simulink model "ADCS_Model"  (R2017b)
settings: Solver=FixedStepAuto  StartTime=0.0  StopTime=10000  FixedStep=1  RelTol=1e-3
libraries: sharedTrackingLibrary x3, simulink x1
settings Model: Creator=caspe  LastModifiedBy=caspe

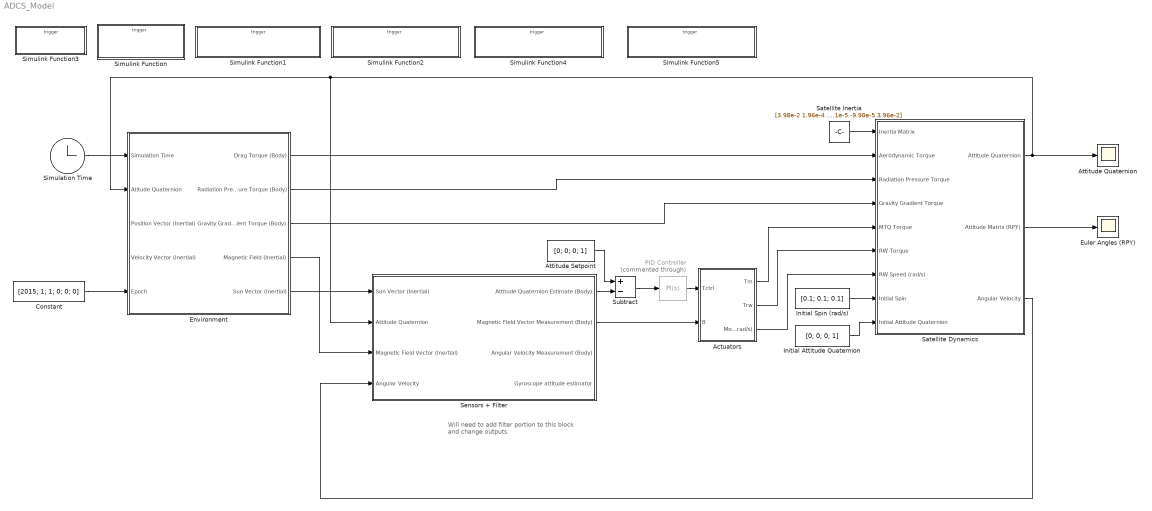
== system ADCS_Model ==
  note: Will need to add filter portion to this block
      | and change outputs.
  Actuators : Subsystem
  Attitude Quaternion : Scope
  Attitude Setpoint : Constant  Value=[0; 0; 0; 1]
  Constant : Constant  Value=[2015; 1; 1; 0; 0; 0]
  Environment : Subsystem
  Euler Angles (RPY) : Scope
  Initial Attitude Quaternion : Constant  Value=[0; 0; 0; 1]
  Initial Spin (rad/s) : Constant  Value=[0.1; 0.1; 0.1]
  PID Controller : simulink/Continuous/PID Controller  Commented=through  Controller=PI  TimeDomain=Continuous-time  SampleTime=-1  IntegratorMethod=Forward Euler  FilterMethod=Forward Euler  Form=Parallel  UseFilter=on  ControllerParametersSource=internal  P=eye(4)  I=eye(4)  D=1.1*eye(4)  N=100  InitialConditionSource=internal  InitialConditionForIntegrator=0  InitialConditionForFilter=0  ExternalReset=none  LimitOutput=off  UpperSaturationLimit=inf  LowerSaturationLimit=-inf  LinearizeAsGain=on  AntiWindupMode=none  Kb=1  TrackingMode=off  Kt=1  PParamMin=[]  PParamMax=[]  IParamMin=[]  IParamMax=[]  DParamMin=[]  DParamMax=[]  NParamMin=[]  NParamMax=[]  KbParamMin=[]  KbParamMax=[]  KtParamMin=[]  KtParamMax=[]  POutMin=[]  POutMax=[]  IOutMin=[]  IOutMax=[]  DOutMin=[]  DOutMax=[]  NOutMin=[]  NOutMax=[]  KbOutMin=[]  KbOutMax=[]  KtOutMin=[]  KtOutMax=[]  IntegratorOutMin=[]  IntegratorOutMax=[]  FilterOutMin=[]  FilterOutMax=[]  SumOutMin=[]  SumOutMax=[]  SumI1OutMin=[]  SumI1OutMax=[]  SumI2OutMin=[]  SumI2OutMax=[]  SumI3OutMin=[]  SumI3OutMax=[]  SumDOutMin=[]  SumDOutMax=[]  SaturationOutMin=[]  SaturationOutMax=[]  IntegratorContinuousStateAttributes=''  IntegratorStateMustResolveToSignalObject=off  IntegratorRTWStateStorageClass=Auto  FilterContinuousStateAttributes=''  FilterStateMustResolveToSignalObject=off  FilterRTWStateStorageClass=Auto  DifferentiatorICPrevScaledInput=0  DifferentiatorOutMin=[]  DifferentiatorOutMax=[]  InitialConditionSetting=State (most efficient)  FilterDiffOutCoefMin=[]  FilterDiffOutCoefMax=[]  SumDenOutMin=[]  SumDenOutMax=[]  SumNumOutMin=[]  SumNumOutMax=[]  ReciprocalOutMin=[]  ReciprocalOutMax=[]  DivideOutMin=[]  DivideOutMax=[]  TunerSelectOption=Transfer Function Based (PID Tuner App)
  Satellite Dynamics : Subsystem
  Satellite Inertia : Constant  Value=[3.98e-2 1.96e-4 2.1e-5; 1.96e-4 7.54e-3 -9.98e-5; 2.1e-5 -9.98e-5 3.96e-2]  VectorParams1D=off
  Sensors + Filter : Subsystem
  Simulation Time : Clock
  Simulink Function : Subsystem  TreatAsAtomicUnit=on
  Simulink Function1 : Subsystem  TreatAsAtomicUnit=on
  Simulink Function2 : Subsystem  TreatAsAtomicUnit=on
  Simulink Function3 : Subsystem  TreatAsAtomicUnit=on
  Simulink Function4 : Subsystem  TreatAsAtomicUnit=on
  Simulink Function5 : Subsystem  TreatAsAtomicUnit=on
  Subtract : Sum  Inputs=+-
  wires:
  Simulation Time/1 -> Environment/1(Simulation Time)
  Environment/4(Magnetic Field (Inertial)) -> Sensors + Filter/3(Magnetic Field Vector (Inertial))
  Environment/5(Sun Vector (Inertial)) -> Sensors + Filter/1(Sun Vector (Inertial))
  Satellite Inertia/1 -> Satellite Dynamics/1(Inertia Matrix)
  Environment/1(Drag Torque (Body)) -> Satellite Dynamics/2(Aerodynamic Torque)
  Environment/2(Radiation Pressure Torque (Body)) -> Satellite Dynamics/3(Radiation Pressure Torque)
  Environment/3(Gravity Gradient Torque (Body)) -> Satellite Dynamics/4(Gravity Gradient Torque)
  Satellite Dynamics/3(Angular Velocity) -> Sensors + Filter/4(Angular Velocity)
  Satellite Dynamics/1(Attitude Quaternion) -> Attitude Quaternion/1, Sensors + Filter/2(Attitude Quaternion), Environment/2(Atitude Quaternion)
  Initial Spin (rad/s)/1 -> Satellite Dynamics/8(Initial Spin)
  Initial Attitude Quaternion/1 -> Satellite Dynamics/9(Initial Attitude Quaternion)
  Constant/1 -> Environment/5(Epoch)
  Satellite Dynamics/2(Attitude Matrix (RPY)) -> Euler Angles (RPY)/1
  Subtract/1 -> PID Controller/1
  Attitude Setpoint/1 -> Subtract/1
  Sensors + Filter/1(Attitude Quaternion Estimate (Body)) -> Subtract/2
  PID Controller/1 -> Actuators/1(Tctrl)
  Sensors + Filter/2(Magnetic Field Vector Measurement (Body)) -> Actuators/2(B)
  Actuators/2(Trw) -> Satellite Dynamics/6(RW Torque)
  Actuators/1(Tm) -> Satellite Dynamics/5(MTQ Torque)
  Actuators/3(Momentum wheel speed (rad/s)) -> Satellite Dynamics/7(RW Speed (rad/s))

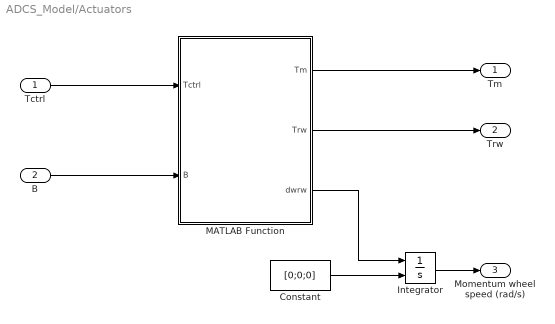
== system ADCS_Model/Actuators ==
  Tctrl : Inport
  B : Inport  Port=2
  Constant : Constant  Value=[0;0;0]
  Integrator : Integrator  InitialConditionSource=external
  MATLAB Function : MATLAB Function  TreatAsAtomicUnit=on
  Tm : Outport
  Trw : Outport  Port=2
  Momentum wheel speed (rad/s) : Outport  Port=3
  wires:
  Tctrl/1 -> MATLAB Function/1(Tctrl)
  B/1 -> MATLAB Function/2(B)
  MATLAB Function/1(Tm) -> Tm/1
  MATLAB Function/2(Trw) -> Trw/1
  MATLAB Function/3(dwrw) -> Integrator/1
  Integrator/1 -> Momentum wheel speed (rad/s)/1
  Constant/1 -> Integrator/2

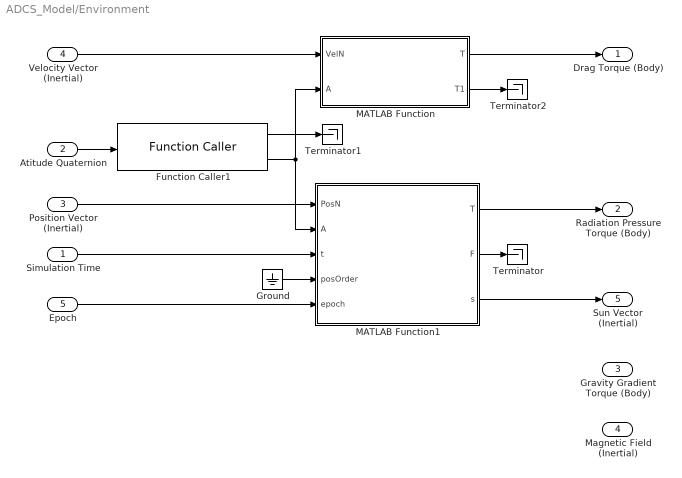
== system ADCS_Model/Environment ==
  Simulation Time : Inport
  Atitude Quaternion : Inport  Port=2
  Position Vector (Inertial) : Inport  Port=3
  Velocity Vector (Inertial) : Inport  Port=4
  Epoch : Inport  Port=5
  Function Caller1 : FunctionCaller  FunctionPrototype=[q,A] = quaternionAttitudeMatrix(x)
  Ground : Ground
  MATLAB Function : MATLAB Function  TreatAsAtomicUnit=on
  MATLAB Function1 : MATLAB Function  TreatAsAtomicUnit=on
  Terminator : Terminator
  Terminator1 : Terminator
  Terminator2 : Terminator
  Drag Torque (Body) : Outport
  Radiation Pressure Torque (Body) : Outport  Port=2
  Gravity Gradient Torque (Body) : Outport  Port=3
  Magnetic Field (Inertial) : Outport  Port=4
  Sun Vector (Inertial) : Outport  Port=5
  wires:
  Velocity Vector (Inertial)/1 -> MATLAB Function/1(VelN)
  Atitude Quaternion/1 -> Function Caller1/1
  Simulation Time/1 -> MATLAB Function1/3(t)
  Position Vector (Inertial)/1 -> MATLAB Function1/1(PosN)
  Function Caller1/1 -> Terminator1/1
  Function Caller1/2 -> MATLAB Function1/2(A), MATLAB Function/2(A)
  MATLAB Function/2(T1) -> Terminator2/1
  MATLAB Function/1(T) -> Drag Torque (Body)/1
  Ground/1 -> MATLAB Function1/4(posOrder)
  Epoch/1 -> MATLAB Function1/5(epoch)
  MATLAB Function1/2(F) -> Terminator/1
  MATLAB Function1/3(s) -> Sun Vector (Inertial)/1
  MATLAB Function1/1(T) -> Radiation Pressure Torque (Body)/1

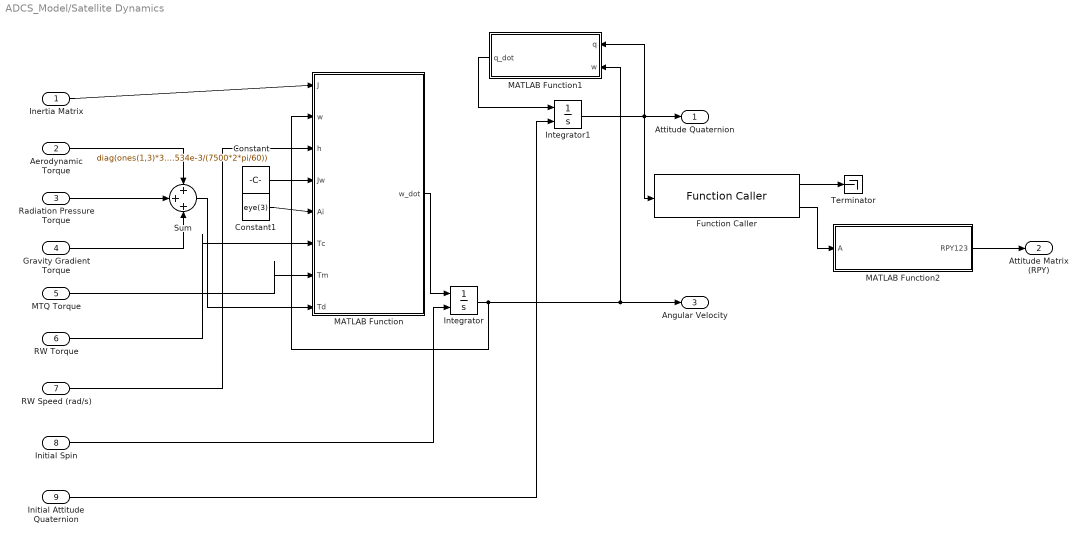
== system ADCS_Model/Satellite Dynamics ==
  Inertia Matrix : Inport
  Aerodynamic Torque : Inport  Port=2
  Radiation Pressure Torque : Inport  Port=3
  Gravity Gradient Torque : Inport  Port=4
  MTQ Torque : Inport  Port=5
  RW Torque : Inport  Port=6
  RW Speed (rad/s) : Inport  Port=7
  Initial Spin : Inport  Port=8
  Initial Attitude Quaternion : Inport  Port=9
  Constant : Constant  Value=diag(ones(1,3)*3.534e-3/(7500*2*pi/60))
  Constant1 : Constant  Value=eye(3)
  Function Caller : FunctionCaller  FunctionPrototype=[q,A] = quaternionAttitudeMatrix(x)
  Integrator : Integrator  InitialConditionSource=external
  Integrator1 : Integrator  InitialConditionSource=external
  MATLAB Function : MATLAB Function  TreatAsAtomicUnit=on
  MATLAB Function1 : MATLAB Function  TreatAsAtomicUnit=on
  MATLAB Function2 : MATLAB Function  TreatAsAtomicUnit=on
  Sum : Sum  Inputs=+++
  Terminator : Terminator
  Attitude Quaternion : Outport
  Attitude Matrix (RPY) : Outport  Port=2
  Angular Velocity : Outport  Port=3
  wires:
  Aerodynamic Torque/1 -> Sum/1
  Radiation Pressure Torque/1 -> Sum/2
  Gravity Gradient Torque/1 -> Sum/3
  RW Torque/1 -> MATLAB Function/6(Tc)
  Integrator/1 -> MATLAB Function/2(w), MATLAB Function1/2(w), Angular Velocity/1
  Initial Spin/1 -> Integrator/2
  MTQ Torque/1 -> MATLAB Function/7(Tm)
  MATLAB Function/1(w_dot) -> Integrator/1
  RW Speed (rad/s)/1 -> MATLAB Function/3(h)
  Inertia Matrix/1 -> MATLAB Function/1(J)
  Sum/1 -> MATLAB Function/8(Td)
  Constant/1 -> MATLAB Function/4(Jw)
  Constant1/1 -> MATLAB Function/5(Ai)
  Initial Attitude Quaternion/1 -> Integrator1/2
  Integrator1/1 -> Function Caller/1, MATLAB Function1/1(q), Attitude Quaternion/1
  MATLAB Function1/1(q_dot) -> Integrator1/1
  Function Caller/1 -> Terminator/1
  Function Caller/2 -> MATLAB Function2/1(A)
  MATLAB Function2/1(RPY123) -> Attitude Matrix (RPY)/1

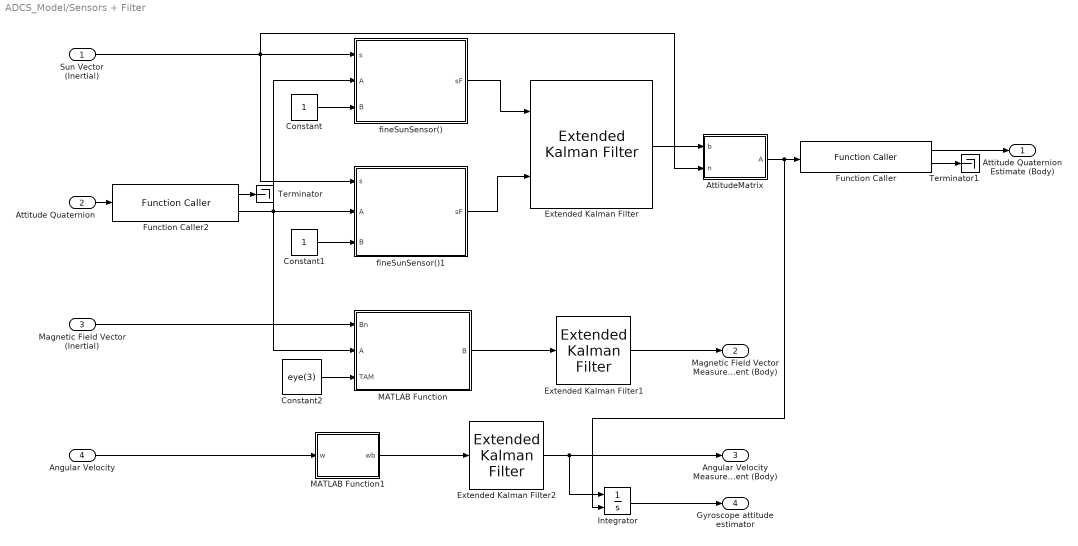
== system ADCS_Model/Sensors + Filter ==
  Sun Vector (Inertial) : Inport
  Attitude Quaternion : Inport  Port=2
  Magnetic Field Vector (Inertial) : Inport  Port=3
  Angular Velocity : Inport  Port=4
  AttitudeMatrix : MATLAB Function  TreatAsAtomicUnit=on
  Constant : Constant
  Constant1 : Constant
  Constant2 : Constant  Value=eye(3)
  Extended Kalman Filter : sharedTrackingLibrary/Extended Kalman Filter  StateTransitionFcn=stateTrans  HasStateTransitionJacobianFcn=off  HasAdditiveProcessNoise=Additive  ProcessNoise=1  HasTimeVaryingProcessNoise=off  HasStateTransitionFcnExtraArgument=0  InitialState=0  InitialStateCovariance=1  MeasurementFcn1=addSunSensorNoise  HasMeasurementJacobianFcn1=off  HasMeasurementEnablePort1=off  HasAdditiveMeasurementNoise1=Additive  MeasurementNoise1=1  HasTimeVaryingMeasurementNoise1=off  HasMeasurementFcnExtraArgument1=0  MeasurementFcn2=addSunSensorNoise  HasMeasurementJacobianFcn2=off  HasMeasurementEnablePort2=off  HasAdditiveMeasurementNoise2=Additive  MeasurementNoise2=1  HasTimeVaryingMeasurementNoise2=off  HasMeasurementFcnExtraArgument2=0  MeasurementFcn3=myMeasurementFcn  HasMeasurementJacobianFcn3=off  HasMeasurementEnablePort3=off  HasAdditiveMeasurementNoise3=Additive  MeasurementNoise3=1  HasTimeVaryingMeasurementNoise3=off  HasMeasurementFcnExtraArgument3=0  MeasurementFcn4=myMeasurementFcn  HasMeasurementJacobianFcn4=off  HasMeasurementEnablePort4=off  HasAdditiveMeasurementNoise4=Additive  MeasurementNoise4=1  HasTimeVaryingMeasurementNoise4=off  HasMeasurementFcnExtraArgument4=0  MeasurementFcn5=myMeasurementFcn  HasMeasurementJacobianFcn5=off  HasMeasurementEnablePort5=off  HasAdditiveMeasurementNoise5=Additive  MeasurementNoise5=1  HasTimeVaryingMeasurementNoise5=off  HasMeasurementFcnExtraArgument5=0  EnableMultirate=off  StateTransitionFcnSampleTime=1  MeasurementFcn1SampleTime=1  MeasurementFcn2SampleTime=1  MeasurementFcn3SampleTime=1  MeasurementFcn4SampleTime=1  MeasurementFcn5SampleTime=1  UseCurrentEstimator=on  OutputStateCovariance=off  DataType=double  SampleTime=1  NumberOfMeasurements=2
      settings: SourceProductName=Control System Toolbox  SourceProductBaseCode=CT
  Extended Kalman Filter1 : sharedTrackingLibrary/Extended Kalman Filter  StateTransitionFcn=stateTrans  HasStateTransitionJacobianFcn=off  HasAdditiveProcessNoise=Additive  ProcessNoise=1  HasTimeVaryingProcessNoise=off  HasStateTransitionFcnExtraArgument=0  InitialState=0  InitialStateCovariance=1  MeasurementFcn1=addTAMNoise  HasMeasurementJacobianFcn1=off  HasMeasurementEnablePort1=off  HasAdditiveMeasurementNoise1=Additive  MeasurementNoise1=1  HasTimeVaryingMeasurementNoise1=off  HasMeasurementFcnExtraArgument1=0  MeasurementFcn2=myMeasurementFcn  HasMeasurementJacobianFcn2=off  HasMeasurementEnablePort2=off  HasAdditiveMeasurementNoise2=Additive  MeasurementNoise2=1  HasTimeVaryingMeasurementNoise2=off  HasMeasurementFcnExtraArgument2=0  MeasurementFcn3=myMeasurementFcn  HasMeasurementJacobianFcn3=off  HasMeasurementEnablePort3=off  HasAdditiveMeasurementNoise3=Additive  MeasurementNoise3=1  HasTimeVaryingMeasurementNoise3=off  HasMeasurementFcnExtraArgument3=0  MeasurementFcn4=myMeasurementFcn  HasMeasurementJacobianFcn4=off  HasMeasurementEnablePort4=off  HasAdditiveMeasurementNoise4=Additive  MeasurementNoise4=1  HasTimeVaryingMeasurementNoise4=off  HasMeasurementFcnExtraArgument4=0  MeasurementFcn5=myMeasurementFcn  HasMeasurementJacobianFcn5=off  HasMeasurementEnablePort5=off  HasAdditiveMeasurementNoise5=Additive  MeasurementNoise5=1  HasTimeVaryingMeasurementNoise5=off  HasMeasurementFcnExtraArgument5=0  EnableMultirate=off  StateTransitionFcnSampleTime=1  MeasurementFcn1SampleTime=1  MeasurementFcn2SampleTime=1  MeasurementFcn3SampleTime=1  MeasurementFcn4SampleTime=1  MeasurementFcn5SampleTime=1  UseCurrentEstimator=on  OutputStateCovariance=off  DataType=double  SampleTime=1  NumberOfMeasurements=1
      settings: SourceProductName=Control System Toolbox  SourceProductBaseCode=CT
  Extended Kalman Filter2 : sharedTrackingLibrary/Extended Kalman Filter  StateTransitionFcn=stateTrans  HasStateTransitionJacobianFcn=off  HasAdditiveProcessNoise=Additive  ProcessNoise=1  HasTimeVaryingProcessNoise=off  HasStateTransitionFcnExtraArgument=0  InitialState=0  InitialStateCovariance=1  MeasurementFcn1=addGyroNoise  HasMeasurementJacobianFcn1=off  HasMeasurementEnablePort1=off  HasAdditiveMeasurementNoise1=Additive  MeasurementNoise1=1  HasTimeVaryingMeasurementNoise1=off  HasMeasurementFcnExtraArgument1=0  MeasurementFcn2=myMeasurementFcn  HasMeasurementJacobianFcn2=off  HasMeasurementEnablePort2=off  HasAdditiveMeasurementNoise2=Additive  MeasurementNoise2=1  HasTimeVaryingMeasurementNoise2=off  HasMeasurementFcnExtraArgument2=0  MeasurementFcn3=myMeasurementFcn  HasMeasurementJacobianFcn3=off  HasMeasurementEnablePort3=off  HasAdditiveMeasurementNoise3=Additive  MeasurementNoise3=1  HasTimeVaryingMeasurementNoise3=off  HasMeasurementFcnExtraArgument3=0  MeasurementFcn4=myMeasurementFcn  HasMeasurementJacobianFcn4=off  HasMeasurementEnablePort4=off  HasAdditiveMeasurementNoise4=Additive  MeasurementNoise4=1  HasTimeVaryingMeasurementNoise4=off  HasMeasurementFcnExtraArgument4=0  MeasurementFcn5=myMeasurementFcn  HasMeasurementJacobianFcn5=off  HasMeasurementEnablePort5=off  HasAdditiveMeasurementNoise5=Additive  MeasurementNoise5=1  HasTimeVaryingMeasurementNoise5=off  HasMeasurementFcnExtraArgument5=0  EnableMultirate=off  StateTransitionFcnSampleTime=1  MeasurementFcn1SampleTime=1  MeasurementFcn2SampleTime=1  MeasurementFcn3SampleTime=1  MeasurementFcn4SampleTime=1  MeasurementFcn5SampleTime=1  UseCurrentEstimator=on  OutputStateCovariance=off  DataType=double  SampleTime=1  NumberOfMeasurements=1
      settings: SourceProductName=Control System Toolbox  SourceProductBaseCode=CT
  Function Caller : FunctionCaller  FunctionPrototype=[q,A] = quaternionAttitudeMatrix(x)
  Function Caller2 : FunctionCaller  FunctionPrototype=[q,A] = quaternionAttitudeMatrix(x)
  Integrator : Integrator  InitialConditionSource=external
  MATLAB Function : MATLAB Function  TreatAsAtomicUnit=on
  MATLAB Function1 : MATLAB Function  TreatAsAtomicUnit=on
  Terminator : Terminator
  Terminator1 : Terminator
  fineSunSensor() : MATLAB Function  TreatAsAtomicUnit=on
  fineSunSensor()1 : MATLAB Function  TreatAsAtomicUnit=on
  Attitude Quaternion Estimate (Body) : Outport
  Magnetic Field Vector Measurement (Body) : Outport  Port=2
  Angular Velocity Measurement (Body) : Outport  Port=3
  Gyroscope attitude estimator : Outport  Port=4
  wires:
  Sun Vector (Inertial)/1 -> fineSunSensor()1/1(s), AttitudeMatrix/2(n), fineSunSensor()/1(s)
  Constant/1 -> fineSunSensor()/3(B)
  Constant1/1 -> fineSunSensor()1/3(B)
  Attitude Quaternion/1 -> Function Caller2/1
  Function Caller2/2 -> MATLAB Function/2(A), fineSunSensor()1/2(A), fineSunSensor()/2(A)
  Magnetic Field Vector (Inertial)/1 -> MATLAB Function/1(Bn)
  Constant2/1 -> MATLAB Function/3(TAM)
  Angular Velocity/1 -> MATLAB Function1/1(w)
  Function Caller2/1 -> Terminator/1
  fineSunSensor()/1(sF) -> Extended Kalman Filter/1
  fineSunSensor()1/1(sF) -> Extended Kalman Filter/2
  MATLAB Function/1(B) -> Extended Kalman Filter1/1
  Extended Kalman Filter1/1 -> Magnetic Field Vector Measurement (Body)/1
  Extended Kalman Filter/1 -> AttitudeMatrix/1(b)
  Function Caller/1 -> Attitude Quaternion Estimate (Body)/1
  Function Caller/2 -> Terminator1/1
  MATLAB Function1/1(wb) -> Extended Kalman Filter2/1
  Extended Kalman Filter2/1 -> Angular Velocity Measurement (Body)/1, Integrator/1
  Integrator/1 -> Gyroscope attitude estimator/1
  AttitudeMatrix/1(A) -> Integrator/2, Function Caller/1

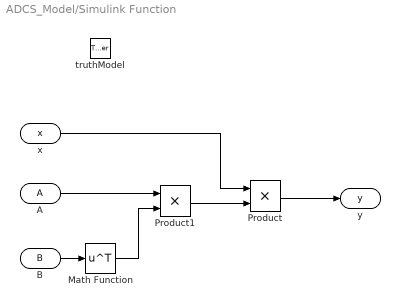
== system ADCS_Model/Simulink Function ==
  truthModel : TriggerPort  TriggerType=function-call  IsSimulinkFunction=on  FunctionName=truthModel  FunctionVisibility=scoped  VariantControl=(inherit)
  Math Function : Math  Operator=transpose  SaturateOnIntegerOverflow=on
  Product : Product
  Product1 : Product
  x : ArgIn  DisableCoverage=on  ArgumentName=x
  A : ArgIn  DisableCoverage=on  Port=2  ArgumentName=A
  B : ArgIn  DisableCoverage=on  Port=3  ArgumentName=B
  y : ArgOut  DisableCoverage=on  ArgumentName=y
  wires:
  Product/1 -> y/1
  Product1/1 -> Product/2
  A/1 -> Product1/1
  B/1 -> Math Function/1
  Math Function/1 -> Product1/2
  x/1 -> Product/1

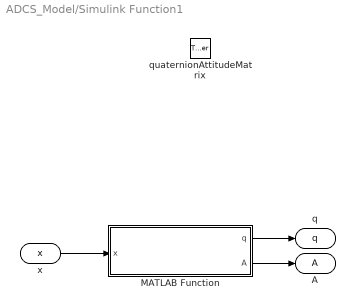
== system ADCS_Model/Simulink Function1 ==
  quaternionAttitudeMatrix : TriggerPort  TriggerType=function-call  IsSimulinkFunction=on  FunctionName=quaternionAttitudeMatrix  FunctionVisibility=scoped  VariantControl=(inherit)
  MATLAB Function : MATLAB Function  TreatAsAtomicUnit=on
  x : ArgIn  DisableCoverage=on  ArgumentName=x
  q : ArgOut  DisableCoverage=on  ArgumentName=q
  A : ArgOut  DisableCoverage=on  Port=2  ArgumentName=A
  wires:
  x/1 -> MATLAB Function/1(x)
  MATLAB Function/1(q) -> q/1
  MATLAB Function/2(A) -> A/1

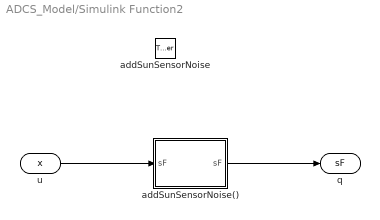
== system ADCS_Model/Simulink Function2 ==
  addSunSensorNoise : TriggerPort  TriggerType=function-call  IsSimulinkFunction=on  FunctionName=addSunSensorNoise  FunctionVisibility=scoped  VariantControl=(inherit)
  addSunSensorNoise() : MATLAB Function  TreatAsAtomicUnit=on
  u : ArgIn  DisableCoverage=on  ArgumentName=x
  q : ArgOut  DisableCoverage=on  ArgumentName=sF
  wires:
  u/1 -> addSunSensorNoise()/1("sF ")
  addSunSensorNoise()/1(sF) -> q/1

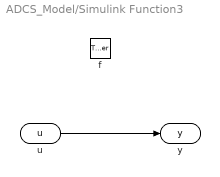
== system ADCS_Model/Simulink Function3 ==
  f : TriggerPort  TriggerType=function-call  IsSimulinkFunction=on  FunctionName=stateTrans  FunctionVisibility=scoped  VariantControl=(inherit)
  u : ArgIn  DisableCoverage=on  ArgumentName=u
  y : ArgOut  DisableCoverage=on  ArgumentName=y
  wires:
  u/1 -> y/1

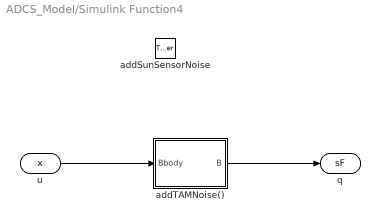
== system ADCS_Model/Simulink Function4 ==
  addSunSensorNoise : TriggerPort  TriggerType=function-call  IsSimulinkFunction=on  FunctionName=addTAMNoise  FunctionVisibility=scoped  VariantControl=(inherit)
  addTAMNoise() : MATLAB Function  TreatAsAtomicUnit=on
  u : ArgIn  DisableCoverage=on  ArgumentName=x
  q : ArgOut  DisableCoverage=on  ArgumentName=sF
  wires:
  u/1 -> addTAMNoise()/1(Bbody)
  addTAMNoise()/1(B) -> q/1

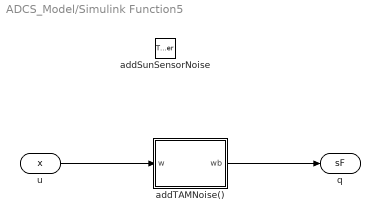
== system ADCS_Model/Simulink Function5 ==
  addSunSensorNoise : TriggerPort  TriggerType=function-call  IsSimulinkFunction=on  FunctionName=addGyroNoise  FunctionVisibility=scoped  VariantControl=(inherit)
  addTAMNoise() : MATLAB Function  TreatAsAtomicUnit=on
  u : ArgIn  DisableCoverage=on  ArgumentName=x
  q : ArgOut  DisableCoverage=on  ArgumentName=sF
  wires:
  u/1 -> addTAMNoise()/1(w)
  addTAMNoise()/1(wb) -> q/1

== matlab function ADCS_Model/Sensors + Filter/fineSunSensor()1 ==
  data: s input; sF output; A input; B input
function sF = fineSunSensor(s, A, B)

% Transform sun vector from inertial to body to fine sun sensor
sF = B'*A*s;
% Check if FSS "sees" sun (FOV +/- 60 deg):
if acosd(dot(sF, [0; 0; 1])) > 180
    sF = zeros(3,1);
else
    % Transform sun vector into sun sensor coordinate system
    % sB = B*sB;
    % Compute sun coordinate angles:
    alpha = acosd(dot(sF, [1; 0; 0]));
    beta = acosd(dot(sF, [0; 1; 0]));
    % Add normally distributed Gaussian noise to angle readings (zero mean,
    % 0.5 degree 3-sigma CI)
    alpha = (0.5/3)*randn(1) + alpha;
    beta = (0.5/3)*randn(1) + beta;
    % Find direction cosines. Gamma dependent on error in alpha and beta.
    calpha = cosd(alpha); cbeta = cosd(beta);
    cgamma = sqrt(1-calpha^2-cbeta^2);
    % Compute sun vector measurement in body-coordinates
    FSS = [calpha; cbeta; cgamma];
    sF = B*FSS;
end
y = u;

== matlab function ADCS_Model/Sensors + Filter/fineSunSensor() ==
  data: s input; sF output; A input; B input
function sF = fineSunSensor(s, A, B)

% Transform sun vector from inertial to body to fine sun sensor
sF = B'*A*s;
% Check if FSS "sees" sun (FOV +/- 60 deg):
if acosd(dot(sF, [0; 0; 1])) > 180
    sF = zeros(3,1);
else
    % Transform sun vector into sun sensor coordinate system
    % sB = B*sB;
    % Compute sun coordinate angles:
    alpha = acosd(dot(sF, [1; 0; 0]));
    beta = acosd(dot(sF, [0; 1; 0]));
    % Add normally distributed Gaussian noise to angle readings (zero mean,
    % 0.5 degree 3-sigma CI)
    alpha = (0.5/3)*randn(1) + alpha;
    beta = (0.5/3)*randn(1) + beta;
    % Find direction cosines. Gamma dependent on error in alpha and beta.
    calpha = cosd(alpha); cbeta = cosd(beta);
    cgamma = sqrt(1-calpha^2-cbeta^2);
    % Compute sun vector measurement in body-coordinates
    FSS = [calpha; cbeta; cgamma];
    sF = B*FSS;
end
y = u;

== matlab function ADCS_Model/Sensors + Filter/AttitudeMatrix ==
  data: b input; A output; n input
function A = fcn(b,n)
if isrow(b)
    b = b';
end
if isrow(n)
    n = n';
end

v = cross(n,b);
s = norm(v);
c = dot(b,n);

A = eye(3) + crossMatrix(v) + (crossMatrix(v))^2*((1-c)/s^2);

== matlab function ADCS_Model/Simulink Function1/MATLAB Function ==
  data: x input; q output; A output
function [q, A] = quaternionAttitudeMatrix(x)

if isvector(x)
    assert(length(x) == 4, 'Quaternion must be 1x4');
    if isrow(x)
        x = x';
    end
    A = Xi(x)'*Psi(x);
    q = x;
else
    assert(mean(size(x)) == 3, 'Direction cosine matrix must be 3x3');
    q = zeros(4,1);
    q(4) = sqrt(1+trace(x))/2;
    q(1) = 1/4/q(4)*(x(2,3)-x(3,2));
    q(2) = 1/4/q(4)*(x(3,1)-x(1,3));
    q(3) = 1/4/q(4)*(x(1,2)-x(2,1));
    A = x;
end
    function [ xi ] = Xi(q)
        q4 = q(4); qbar = q(1:3);
        xi = [q4*eye(3)+crossMatrix(qbar); -qbar'];
    end
    function [ psi ] = Psi(q)
        q4 = q(4); qbar = q(1:3);
        psi = [q4*eye(3)-crossMatrix(qbar); -qbar'];
    end
end

== matlab function ADCS_Model/Simulink Function2/addSunSensorNoise() ==
  data: sF input; sF output
function sF = fcn(sF)

% Check if FSS "sees" sun (FOV +/- 60 deg):
if acosd(dot(sF, [0; 0; 1])) > 180
    sF = zeros(3,1);
else
    % Transform sun vector into sun sensor coordinate system
    % sB = B*sB;
    % Compute sun coordinate angles:
    alpha = acosd(dot(sF, [1; 0; 0]));
    beta = acosd(dot(sF, [0; 1; 0]));
    % Add normally distributed Gaussian noise to angle readings (zero mean,
    % 0.5 degree 3-sigma CI)
    alpha = (0.5/3)*randn(1) + alpha;
    beta = (0.5/3)*randn(1) + beta;
    % Find direction cosines. Gamma dependent on error in alpha and beta.
    calpha = cosd(alpha); cbeta = cosd(beta);
    cgamma = sqrt(1-calpha^2-cbeta^2);
    % Compute sun vector measurement in body-coordinates
    FSS = [calpha; cbeta; cgamma];
    sF = B*FSS;
end

== matlab function ADCS_Model/Simulink Function4/addTAMNoise() ==
  data: Bbody input; B output
function B = fcn(Bbody)

% Noise parameters: accuracy and associated confidence interval
accuracy = []; sigma = []; 
% Add noise to local magnetic field value for sensor output
B = (accuracy/sigma)*randn(3,1) + Bbody;
end

== matlab function ADCS_Model/Environment/MATLAB Function ==
  data: VelN input; T output; A input; T1 output
function [T, T1] = aerodynDrag(VelN, A)

% Make sure VelN is a column vector
if ~iscolumn(VelN)
    VelN = VelN';
end

% Atmospheric density at 400km altitude per the MSISE-90 Model of Earth's
% Upper Atmosphere (kg m^-3)
LowActivityDensity = 5.68e-13; HighActivityDensity = 5.04e-11;
% Assign local density a psuedorandom value on the interval of low solar
% activity density to hihgh solar activity density (kg m^-3). Can update
% this to resemble a Gaussian distribution.
rho = LowActivityDensity + (HighActivityDensity - LowActivityDensity)...
    *randn(1);
% Define momentum transfer coefficients
s_n = 0.5; s_t = 0.5;
% Surface areas of sides of CubeSat; Area vector
A_3U = 0.3*0.1; A_1U = 0.1*0.1; 
surf = [A_1U, A_3U, A_3U]; surf = [surf, surf];
% Create velocity unit vector and velocity magnitude in body coordinates
V = norm(VelN); e_v = A*(VelN/V);
% Create check for frontal areas of the satellite (c > 0)
e_vBdot = [e_v, e_v, e_v, e_v, e_v, e_v]';
Bni = [1 0 0; 0 1 0; 0 0 1; -1 0 0; 0 -1 0; 0 0 -1];
c = dot(Bni, e_vBdot, 2);
% Calculate aerodynamic drag force
F = 0;
for i = 1:6
    if c(i) > 0
        F = F + (-rho*V^2*((2-s_n-s_t)*(dot(e_v, Bni(i,:)))^2*Bni(i,:)'+...
            s_t*(dot(e_v, Bni(i,:)))*e_v)*surf(i));
    end
end
% Add 10% pseudorandom variation to the force vector due to uncertainty
% in solar pressure value, optical behavior, and moment arm to center
% of pressure
F = (0.9 + (1.1-0.9)*randn(3,1)).*F;
% Define center of pressure moment arm r, and the aerodynamic disturbance 
% torque T as the cross product rxF, all in body coordinates
r = [0.01; 0.01; 0.01];
T = cross(r,F);

== matlab function ADCS_Model/Environment/MATLAB Function1 ==
  data: PosN input; T output; A input; t input; posOrder input; epoch input; F output; s output
function [T, F, s] = solarRadPress(PosN, A, t, posOrder, epoch)

if strcmp(posOrder, 'sphere')
    PosN = sph2cart(PosN(1), PosN(2), PosN(3));
elseif strcmp(posOrder, 'cylin')
    PosN = pol2cart(PosN(1), PosN(2), PosN(3));
end

% Specular reflection and diffusion coefficients for each of the six
% surfaces of a CubeSat. Surface property. (unitless in [0,1]) Current
% values are speculative.
Rspec = 0.6; Rspec = Rspec.*ones(1,6); 
Rdiff = 0.2; Rdiff = Rdiff.*ones(1,6);
% Surface areas of sides of CubeSat; Area vector
A_3U = 0.3*0.1; A_1U = 0.1*0.1; 
surf = [A_1U, A_3U, A_3U]; surf = [surf, surf];
% Get sun vector in inertial coordinates
[s, Rs] = sunVec(PosN, t, posOrder, epoch);
% Transform sun vector to body coordinates
sB = A*s;
% Create check for which sides of the satellite can be "seen" (c > 0)
sBdot = [sB, sB, sB, sB, sB, sB]';
Bni = [1 0 0; 0 1 0; 0 0 1; -1 0 0; 0 -1 0; 0 0 -1];
c = dot(Bni, sBdot, 2);
% Solar radiation intensity variation, given a 5% pseudorandom uncertainty 
% fluctuation to account for solar activity and uncertainty in the
% parameter. Distance values must be in terms of AU.
Rs = s*Rs; R = Rs-(PosN./149597870700);
P = (1362/(299792458*norm(R)^2))*(0.95 + (1.05-0.95)*randn(1));
% Calculate solar pressure force
F = 0;
for i = 1:6
    if c(i) > 0
        F = F + (-P*surf(i)*c(i)*(2*(Rdiff(i)/3+Rspec(i)*c(i))*...
            (A'*Bni(i,:)')+(1-Rspec(i))*sB));
    end
end
% Add 10% pseudorandom variation to the force vector due to uncertainty
% in solar pressure value, optical behavior, and moment arm to center
% of pressure
F = (0.9 + (1.1-0.9)*randn(3,1)).*F;
% Define center of pressure moment arm r, and the radiation pressure 
% torque T as the cross product rxF, all in body coordinates
r = [0.01; 0.01; 0.01];
T = cross(r,F);

== matlab function ADCS_Model/Sensors + Filter/MATLAB Function ==
  data: Bn input; B output; A input; TAM input
function B   = threeAxisMagnetometer( Bn, A, TAM )
% threeAxisMagnetometer    Produces magnetometer sensor reading from model
%   
%   [B] = threeAxisMagnetometer(Bn, A, TAM) will return the output of a
%   magnetometer given a model magnetic field vector Bn in inertial 
%   coordinates. The output vector B will be in the body-coordinate system.
%   The matrix TAM (optional) is a rotation matrix that transforms the 
%   axes of the satellite to that of the magnetometer, if it is tilted 
%   off-axis. If TAM is not set, it will be assumed TAM = eye(3).
%
%   For the matrix TAM, the third column should contain the coordinates 
%   for the vector perpendicular to the sensor of the magnetometer, 
%   defined in the body coordinate frame. The coordinates defined by the 
%   matrix B should be orthogonal.
%
%   Class support for inputs s, A, B
%     float: double, single

if nargin < 3
    TAM = eye(3);
    if nargin < 2
        error(message('MATLAB:narginchk:notEnoughInputs'));
    end
end

% Transform magnetic field vector from inertial to body to magnetometer
Bbody = TAM'*A*Bn;
% Noise parameters: accuracy and associated confidence interval
accuracy = []; sigma = []; 
% Add noise to local magnetic field value for sensor output
B = (accuracy/sigma)*randn(3,1) + Bbody;

end

== matlab function ADCS_Model/Satellite Dynamics/MATLAB Function ==
  data: J input; w_dot output; w input; h input; Jw input; Ai input; Tc input; Tm input; Td input
function w_dot = satelliteDynamics(J, w, h, Jw, Ai, Tc, Tm, Td)

J_hat = J-(Ai*Jw)*Ai';
w_dot = J_hat\(-crossMatrix(w)*(J*w+Ai*Jw*h)+Ai*Tc+Tm+Td);

== matlab function ADCS_Model/Satellite Dynamics/MATLAB Function1 ==
  data: q input; q_dot output; w input
function q_dot = quaternionRate(q, w)

q4 = q(4);

q_dot = [q4*eye(3)+crossmatrix(q(1:3)); -q(1:3)']/2*w;

== matlab function ADCS_Model/Satellite Dynamics/MATLAB Function2 ==
  data: A input; RPY123 output
function RPY123 = attitudeMatrix2RPY123(A)

roll_phi = -atand(A(3,2)/A(3,3));
pitch_theta = asind(A(3,1));
yaw_psi = -atand(A(2,1)/A(1,1));

RPY123 = [roll_phi; pitch_theta; yaw_psi];
end

== matlab function ADCS_Model/Sensors + Filter/MATLAB Function1 ==
  data: w input; wb output
function wb   = gyroscope( w ) 
%gyroscope      Gyroscope angular velocity reading
%
%   [wb] = gyroscope(w) will produce the body-coordinate angular velocity
%   vector 'wb' by adding gyro bias and gaussian noise to the model angular
%   velocity vector 'w'. 
%
%   [wb, t] = gyroscope(w) will also output the orientation change due to
%   the angular velocity vector 'wb' in 't'. The output 't' will be
%   calculated from 'wb' to account for gyroscopic drift in the sensor
%   reading.
%
%   Class support for input w
%     float: double, single

if nargin < 1
    error(message('MATLAB:narginchk:notEnoughInputs'));
end

% Define sensor bias and noise parameters
bias = []; accuracy = []; sigma = [];
wb = (accuracy/sigma)*randn(3,1)+bias+w;

end

== matlab function ADCS_Model/Simulink Function5/addTAMNoise() ==
  data: w input; wb output
function wb   = gyroscopeN( w ) 
%gyroscope      Gyroscope angular velocity reading
%
%   [wb] = gyroscope(w) will produce the body-coordinate angular velocity
%   vector 'wb' by adding gyro bias and gaussian noise to the model angular
%   velocity vector 'w'. 
%
%   [wb, t] = gyroscope(w) will also output the orientation change due to
%   the angular velocity vector 'wb' in 't'. The output 't' will be
%   calculated from 'wb' to account for gyroscopic drift in the sensor
%   reading.
%
%   Class support for input w
%     float: double, single

if nargin < 1
    error(message('MATLAB:narginchk:notEnoughInputs'));
end

% Define sensor bias and noise parameters
bias = []; accuracy = []; sigma = [];
wb = (accuracy/sigma)*randn(3,1)+bias+w;

end

== matlab function ADCS_Model/Actuators/MATLAB Function ==
  data: Tctrl input; Tm output; B input; Trw output; dwrw output
function [ Tm, Trw, dwrw ] = actuatorModel( Tctrl, B)

mu = cross(Tctrl, B);
musat = 0.015;
if max(mu) <= musat
    mu_m = mu;
else
    mu_unit = mu/norm(mu);
    mu_max = max(mu);T
    mu_m = musat/mu_max*mu_unit;
end
Tm = cross(mu_m, B);

Trem = Tctrl - Tm;
if Trem == zeros(3,1)
    
Irw = 3.534e-3/(7500*2*pi/60);
dwrw = Trem/Irw; 
%somehow cap the increase in reaction wheel speed

wrw_new = wrw+dwrw;
Trw = Irw*dwrw;

end

end
